simulink model "Feedforward_compensation_control"  (R2016a)
settings: Solver=VariableStepAuto  StartTime=0.0  StopTime=100  RelTol=1e-3
values from neighbouring files (symbols this model uses):
  K1 = 1    [initial_composite_control.m]    (also in initial_feedforward_compensation_control.m; initial_speed_measurement_feedback.m = 100)
  Km = 1    [initial_feedforward_compensation_control.m]
  Kn = 1    [initial_feedforward_compensation_control.m]
  T1 = 1    [initial_composite_control.m]    (also in initial_feedforward_compensation_control.m)
  T2 = 1    [initial_composite_control.m]    (also in initial_feedforward_compensation_control.m = 0.01)
  Tm = 1    [initial_feedforward_compensation_control.m]
libraries: simulink x2
settings Model: Creator=73565  LastModifiedBy=73565

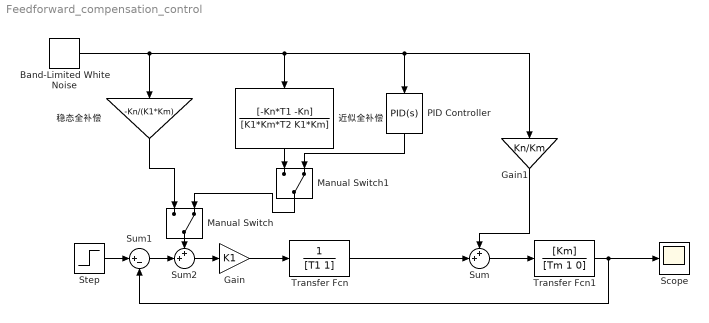
== system Feedforward_compensation_control ==
  Band-Limited White Noise : simulink/Sources/Band-Limited White Noise  Cov=[0.1]  Ts=0.1  seed=[23341]
  Gain : Gain  Gain=K1
  Gain1 : Gain  Gain=Kn/Km
  Manual Switch : ManualSwitch  CurrentSetting=0
  Manual Switch1 : ManualSwitch  CurrentSetting=0
  PID Controller : simulink/Continuous/PID Controller  Controller=PID  TimeDomain=Continuous-time  SampleTime=-1  IntegratorMethod=Forward Euler  FilterMethod=Forward Euler  Form=Parallel  UseFilter=on  ControllerParametersSource=internal  P=-Kn*T1/(K1*Km)  I=0  D=-Kn/(K1*Km)  N=100  InitialConditionSource=internal  InitialConditionForIntegrator=0  InitialConditionForFilter=0  ExternalReset=none  LimitOutput=off  UpperSaturationLimit=inf  LowerSaturationLimit=-inf  LinearizeAsGain=on  AntiWindupMode=none  Kb=1  TrackingMode=off  Kt=1  PParamMin=[]  PParamMax=[]  IParamMin=[]  IParamMax=[]  DParamMin=[]  DParamMax=[]  NParamMin=[]  NParamMax=[]  KbParamMin=[]  KbParamMax=[]  KtParamMin=[]  KtParamMax=[]  POutMin=[]  POutMax=[]  IOutMin=[]  IOutMax=[]  DOutMin=[]  DOutMax=[]  NOutMin=[]  NOutMax=[]  KbOutMin=[]  KbOutMax=[]  KtOutMin=[]  KtOutMax=[]  IntegratorOutMin=[]  IntegratorOutMax=[]  FilterOutMin=[]  FilterOutMax=[]  SumOutMin=[]  SumOutMax=[]  SumI1OutMin=[]  SumI1OutMax=[]  SumI2OutMin=[]  SumI2OutMax=[]  SumI3OutMin=[]  SumI3OutMax=[]  SumDOutMin=[]  SumDOutMax=[]  SaturationOutMin=[]  SaturationOutMax=[]  IntegratorContinuousStateAttributes=''  IntegratorStateMustResolveToSignalObject=off  IntegratorRTWStateStorageClass=Auto  FilterContinuousStateAttributes=''  FilterStateMustResolveToSignalObject=off  FilterRTWStateStorageClass=Auto  DifferentiatorICPrevScaledInput=0  DifferentiatorOutMin=[]  DifferentiatorOutMax=[]
  Scope : Scope
  Step : Step  SampleTime=0
  Sum : Sum  Inputs=++|
  Sum1 : Sum  Inputs=|+-
  Sum2 : Sum  Inputs=++|
  Transfer Fcn : TransferFcn  Denominator=[T1 1]
  Transfer Fcn1 : TransferFcn  Numerator=[Km]  Denominator=[Tm 1 0]
  稳态全补偿 : Gain  Gain=-Kn/(K1*Km)
  近似全补偿 : TransferFcn  Numerator=[-Kn*T1 -Kn]  Denominator=[K1*Km*T2 K1*Km]
  wires:
  Gain/1 -> Transfer Fcn/1
  Transfer Fcn/1 -> Sum/2
  Sum/1 -> Transfer Fcn1/1
  Step/1 -> Sum1/1
  Transfer Fcn1/1 -> Scope/1, Sum1/2
  Gain1/1 -> Sum/1
  Band-Limited White Noise/1 -> PID Controller/1, Gain1/1, 近似全补偿/1, 稳态全补偿/1
  Sum1/1 -> Sum2/2
  Sum2/1 -> Gain/1
  稳态全补偿/1 -> Manual Switch/1
  Manual Switch/1 -> Sum2/1
  近似全补偿/1 -> Manual Switch1/1
  Manual Switch1/1 -> Manual Switch/2
  PID Controller/1 -> Manual Switch1/2
